simulink model "untitled"  (R2025a)
settings: Solver=VariableStepAuto  StartTime=0.0  StopTime=600  RelTol=1e-3  AbsTol=1e-3  EnableMultiTasking=on
libraries: fl_lib x60, nesl_utility x23, ee_lib x14, slpidlib x4, batteryecm_lib x1, simulink x1
(part 2 of 2)

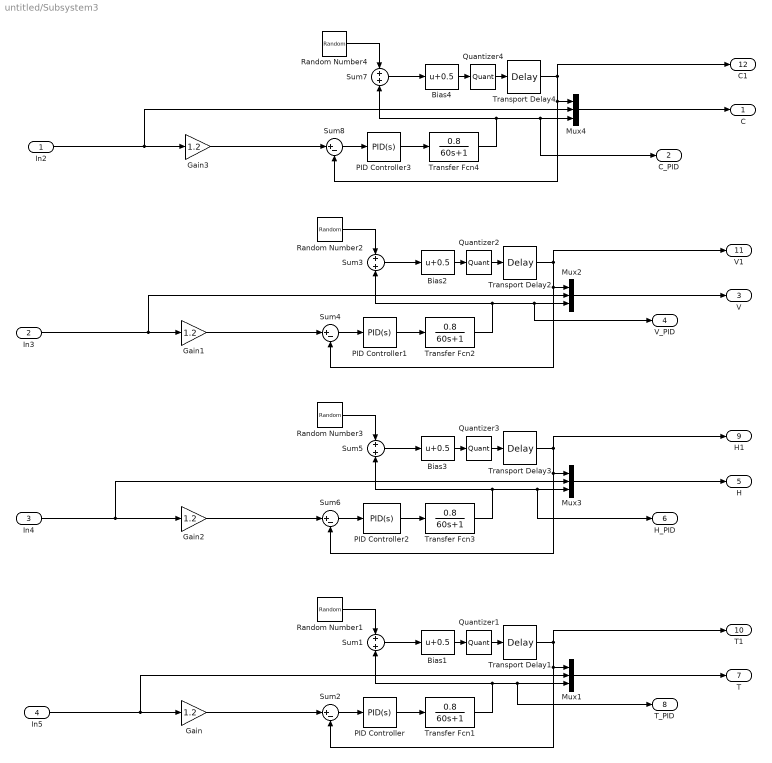
== system untitled/Subsystem3 ==
  In2 : Inport
  In3 : Inport  Port=2
  In4 : Inport  Port=3
  In5 : Inport  Port=4
  Bias{1..4} (4 alike) : Bias  Bias=0.5
  Gain{,1..3} (4 alike) : Gain  Gain=1.2
  Mux{1..4} (4 alike) : Mux  Inputs=3
  PID Controller : slpidlib/PID Controller  Controller=PID  Form=Parallel  TimeDomain=Continuous-time  UseExternalTs=off  SampleTime=-1  IntegratorMethod=Forward Euler  FilterMethod=Forward Euler  ControllerParametersSource=internal  P=2.12001784714755  I=0.0555587280074355  UseKiTs=off  D=0  UseExternalDerivativeSource=off  N=0.0353057614691729  UseFilter=on  TunerSelectOption=Transfer Function Based (PID Tuner App)  InitialConditionSource=internal  InitialConditionForIntegrator=0  InitialConditionForFilter=0  DifferentiatorICPrevScaledInput=0  ExternalReset=none  TrackingMode=off  Kt=1  LimitOutput=off  SatLimitsSource=internal  UpperSaturationLimit=inf  LowerSaturationLimit=-inf  LinearizeAsGain=on  AntiWindupMode=none  Kb=1  LimitIntegrator=off  UpperIntegratorSaturationLimit=inf  LowerIntegratorSaturationLimit=-inf  POutMin=[]  POutMax=[]  IOutMin=[]  IOutMax=[]  DOutMin=[]  DOutMax=[]  NOutMin=[]  NOutMax=[]  SumOutMin=[]  SumOutMax=[]  SaturationOutMin=[]  SaturationOutMax=[]  PParamMin=[]  PParamMax=[]  IParamMin=[]  IParamMax=[]  DParamMin=[]  DParamMax=[]  NParamMin=[]  NParamMax=[]  KbParamMin=[]  KbParamMax=[]  KtParamMin=[]  KtParamMax=[]  KbOutMin=[]  KbOutMax=[]  KtOutMin=[]  KtOutMax=[]  IntegratorOutMin=[]  IntegratorOutMax=[]  FilterOutMin=[]  FilterOutMax=[]  SumI1OutMin=[]  SumI1OutMax=[]  SumI2OutMin=[]  SumI2OutMax=[]  SumI3OutMin=[]  SumI3OutMax=[]  SumI4OutMin=[]  SumI4OutMax=[]  SumDOutMin=[]  SumDOutMax=[]  DifferentiatorOutMin=[]  DifferentiatorOutMax=[]  FilterDiffOutCoefMin=[]  FilterDiffOutCoefMax=[]  ReciprocalOutMin=[]  ReciprocalOutMax=[]  SumDenOutMin=[]  SumDenOutMax=[]  SumNumOutMin=[]  SumNumOutMax=[]  DivideOutMin=[]  DivideOutMax=[]  UdiffTsProdOutMin=[]  UdiffTsProdOutMax=[]  NTsProdOutMin=[]  NTsProdOutMax=[]  UintegralTsProdOutMin=[]  UintegralTsProdOutMax=[]  UngainTsProdOutMin=[]  UngainTsProdOutMax=[]  ClampingZeroOutDataTypeStr=Inherit: Inherit via back propagation  ClampingZeroOutMin=[]  ClampingZeroOutMax=[]  FilterDenConstantOutDataTypeStr=Inherit: Inherit via back propagation  FilterDenConstantOutMin=[]  FilterDenConstantOutMax=[]  PCopyOutDataTypeStr=Inherit: Inherit via back propagation  PCopyOutMin=[]  PCopyOutMax=[]  NCopyOutDataTypeStr=Inherit: Inherit via back propagation  NCopyOutMin=[]  NCopyOutMax=[]  IntegratorContinuousStateAttributes=''  IntegratorStateMustResolveToSignalObject=off  IntegratorRTWStateStorageClass=Auto  FilterContinuousStateAttributes=''  FilterStateMustResolveToSignalObject=off  FilterRTWStateStorageClass=Auto  ParallelPVariant=InternalParameters  IdealPVariant=Disabled  IVariant=InternalParameters  DVariant=InternalParameters  IntegratorVariant=Continuous  SatVariant=Disabled  AWVariant=Passthrough  PCopyVariant=Disabled  TRVariant=Disabled  FdbkBlocksVariant=Forward  IdealPFdbkVariant=Disabled  SatFdbkVariant=Disabled  DerivativeFilterVariant=ContFilter  NVariant=InternalParameters  NCopyVariant=Disabled  FilterICVariant=InternalICsFilter  IntegratorICVariant=InternalICs  ExternalResetVariant=Disabled  TRSumVariant=Passthrough  SumFdbkVariant=Disabled  SumVariant=Sum_PID  TsampFilterVariant=InternalTs  TsampNgainVariant=Passthrough  TsampIntegralVariant=Disabled_SignalSpec  ExternalSaturationOutDataTypeStr=Inherit: Same as second input  DerivativeSourceVariant=ErrorSignal  PreIntVariant=InternalPreInt
  PID Controller1 : slpidlib/PID Controller  Controller=PID  Form=Parallel  TimeDomain=Continuous-time  UseExternalTs=off  SampleTime=-1  IntegratorMethod=Forward Euler  FilterMethod=Forward Euler  ControllerParametersSource=internal  P=2.12001784714755  I=0.0555587280074355  UseKiTs=off  D=0  UseExternalDerivativeSource=off  N=100  UseFilter=on  TunerSelectOption=Transfer Function Based (PID Tuner App)  InitialConditionSource=internal  InitialConditionForIntegrator=0  InitialConditionForFilter=0  DifferentiatorICPrevScaledInput=0  ExternalReset=none  TrackingMode=off  Kt=1  LimitOutput=off  SatLimitsSource=internal  UpperSaturationLimit=inf  LowerSaturationLimit=-inf  LinearizeAsGain=on  AntiWindupMode=none  Kb=1  LimitIntegrator=off  UpperIntegratorSaturationLimit=inf  LowerIntegratorSaturationLimit=-inf  POutMin=[]  POutMax=[]  IOutMin=[]  IOutMax=[]  DOutMin=[]  DOutMax=[]  NOutMin=[]  NOutMax=[]  SumOutMin=[]  SumOutMax=[]  SaturationOutMin=[]  SaturationOutMax=[]  PParamMin=[]  PParamMax=[]  IParamMin=[]  IParamMax=[]  DParamMin=[]  DParamMax=[]  NParamMin=[]  NParamMax=[]  KbParamMin=[]  KbParamMax=[]  KtParamMin=[]  KtParamMax=[]  KbOutMin=[]  KbOutMax=[]  KtOutMin=[]  KtOutMax=[]  IntegratorOutMin=[]  IntegratorOutMax=[]  FilterOutMin=[]  FilterOutMax=[]  SumI1OutMin=[]  SumI1OutMax=[]  SumI2OutMin=[]  SumI2OutMax=[]  SumI3OutMin=[]  SumI3OutMax=[]  SumI4OutMin=[]  SumI4OutMax=[]  SumDOutMin=[]  SumDOutMax=[]  DifferentiatorOutMin=[]  DifferentiatorOutMax=[]  FilterDiffOutCoefMin=[]  FilterDiffOutCoefMax=[]  ReciprocalOutMin=[]  ReciprocalOutMax=[]  SumDenOutMin=[]  SumDenOutMax=[]  SumNumOutMin=[]  SumNumOutMax=[]  DivideOutMin=[]  DivideOutMax=[]  UdiffTsProdOutMin=[]  UdiffTsProdOutMax=[]  NTsProdOutMin=[]  NTsProdOutMax=[]  UintegralTsProdOutMin=[]  UintegralTsProdOutMax=[]  UngainTsProdOutMin=[]  UngainTsProdOutMax=[]  ClampingZeroOutDataTypeStr=Inherit: Inherit via back propagation  ClampingZeroOutMin=[]  ClampingZeroOutMax=[]  FilterDenConstantOutDataTypeStr=Inherit: Inherit via back propagation  FilterDenConstantOutMin=[]  FilterDenConstantOutMax=[]  PCopyOutDataTypeStr=Inherit: Inherit via back propagation  PCopyOutMin=[]  PCopyOutMax=[]  NCopyOutDataTypeStr=Inherit: Inherit via back propagation  NCopyOutMin=[]  NCopyOutMax=[]  IntegratorContinuousStateAttributes=''  IntegratorStateMustResolveToSignalObject=off  IntegratorRTWStateStorageClass=Auto  FilterContinuousStateAttributes=''  FilterStateMustResolveToSignalObject=off  FilterRTWStateStorageClass=Auto  ParallelPVariant=InternalParameters  IdealPVariant=Disabled  IVariant=InternalParameters  DVariant=InternalParameters  IntegratorVariant=Continuous  SatVariant=Disabled  AWVariant=Passthrough  PCopyVariant=Disabled  TRVariant=Disabled  FdbkBlocksVariant=Forward  IdealPFdbkVariant=Disabled  SatFdbkVariant=Disabled  DerivativeFilterVariant=ContFilter  NVariant=InternalParameters  NCopyVariant=Disabled  FilterICVariant=InternalICsFilter  IntegratorICVariant=InternalICs  ExternalResetVariant=Disabled  TRSumVariant=Passthrough  SumFdbkVariant=Disabled  SumVariant=Sum_PID  TsampFilterVariant=InternalTs  TsampNgainVariant=Passthrough  TsampIntegralVariant=Disabled_SignalSpec  ExternalSaturationOutDataTypeStr=Inherit: Same as second input  DerivativeSourceVariant=ErrorSignal  PreIntVariant=InternalPreInt
  PID Controller2 : slpidlib/PID Controller  Controller=PID  Form=Parallel  TimeDomain=Continuous-time  UseExternalTs=off  SampleTime=-1  IntegratorMethod=Forward Euler  FilterMethod=Forward Euler  ControllerParametersSource=internal  P=2.12001784714755  I=0.0555587280074355  UseKiTs=off  D=0  UseExternalDerivativeSource=off  N=100  UseFilter=on  TunerSelectOption=Transfer Function Based (PID Tuner App)  InitialConditionSource=internal  InitialConditionForIntegrator=0  InitialConditionForFilter=0  DifferentiatorICPrevScaledInput=0  ExternalReset=none  TrackingMode=off  Kt=1  LimitOutput=off  SatLimitsSource=internal  UpperSaturationLimit=inf  LowerSaturationLimit=-inf  LinearizeAsGain=on  AntiWindupMode=none  Kb=1  LimitIntegrator=off  UpperIntegratorSaturationLimit=inf  LowerIntegratorSaturationLimit=-inf  POutMin=[]  POutMax=[]  IOutMin=[]  IOutMax=[]  DOutMin=[]  DOutMax=[]  NOutMin=[]  NOutMax=[]  SumOutMin=[]  SumOutMax=[]  SaturationOutMin=[]  SaturationOutMax=[]  PParamMin=[]  PParamMax=[]  IParamMin=[]  IParamMax=[]  DParamMin=[]  DParamMax=[]  NParamMin=[]  NParamMax=[]  KbParamMin=[]  KbParamMax=[]  KtParamMin=[]  KtParamMax=[]  KbOutMin=[]  KbOutMax=[]  KtOutMin=[]  KtOutMax=[]  IntegratorOutMin=[]  IntegratorOutMax=[]  FilterOutMin=[]  FilterOutMax=[]  SumI1OutMin=[]  SumI1OutMax=[]  SumI2OutMin=[]  SumI2OutMax=[]  SumI3OutMin=[]  SumI3OutMax=[]  SumI4OutMin=[]  SumI4OutMax=[]  SumDOutMin=[]  SumDOutMax=[]  DifferentiatorOutMin=[]  DifferentiatorOutMax=[]  FilterDiffOutCoefMin=[]  FilterDiffOutCoefMax=[]  ReciprocalOutMin=[]  ReciprocalOutMax=[]  SumDenOutMin=[]  SumDenOutMax=[]  SumNumOutMin=[]  SumNumOutMax=[]  DivideOutMin=[]  DivideOutMax=[]  UdiffTsProdOutMin=[]  UdiffTsProdOutMax=[]  NTsProdOutMin=[]  NTsProdOutMax=[]  UintegralTsProdOutMin=[]  UintegralTsProdOutMax=[]  UngainTsProdOutMin=[]  UngainTsProdOutMax=[]  ClampingZeroOutDataTypeStr=Inherit: Inherit via back propagation  ClampingZeroOutMin=[]  ClampingZeroOutMax=[]  FilterDenConstantOutDataTypeStr=Inherit: Inherit via back propagation  FilterDenConstantOutMin=[]  FilterDenConstantOutMax=[]  PCopyOutDataTypeStr=Inherit: Inherit via back propagation  PCopyOutMin=[]  PCopyOutMax=[]  NCopyOutDataTypeStr=Inherit: Inherit via back propagation  NCopyOutMin=[]  NCopyOutMax=[]  IntegratorContinuousStateAttributes=''  IntegratorStateMustResolveToSignalObject=off  IntegratorRTWStateStorageClass=Auto  FilterContinuousStateAttributes=''  FilterStateMustResolveToSignalObject=off  FilterRTWStateStorageClass=Auto  ParallelPVariant=InternalParameters  IdealPVariant=Disabled  IVariant=InternalParameters  DVariant=InternalParameters  IntegratorVariant=Continuous  SatVariant=Disabled  AWVariant=Passthrough  PCopyVariant=Disabled  TRVariant=Disabled  FdbkBlocksVariant=Forward  IdealPFdbkVariant=Disabled  SatFdbkVariant=Disabled  DerivativeFilterVariant=ContFilter  NVariant=InternalParameters  NCopyVariant=Disabled  FilterICVariant=InternalICsFilter  IntegratorICVariant=InternalICs  ExternalResetVariant=Disabled  TRSumVariant=Passthrough  SumFdbkVariant=Disabled  SumVariant=Sum_PID  TsampFilterVariant=InternalTs  TsampNgainVariant=Passthrough  TsampIntegralVariant=Disabled_SignalSpec  ExternalSaturationOutDataTypeStr=Inherit: Same as second input  DerivativeSourceVariant=ErrorSignal  PreIntVariant=InternalPreInt
  PID Controller3 : slpidlib/PID Controller  Controller=PID  Form=Parallel  TimeDomain=Continuous-time  UseExternalTs=off  SampleTime=-1  IntegratorMethod=Forward Euler  FilterMethod=Forward Euler  ControllerParametersSource=internal  P=2.12001784714755  I=0.0425233068957785  UseKiTs=off  D=8.52577757434395  UseExternalDerivativeSource=off  N=0.0510689208285348  UseFilter=on  TunerSelectOption=Transfer Function Based (PID Tuner App)  InitialConditionSource=internal  InitialConditionForIntegrator=0  InitialConditionForFilter=0  DifferentiatorICPrevScaledInput=0  ExternalReset=none  TrackingMode=off  Kt=1  LimitOutput=off  SatLimitsSource=internal  UpperSaturationLimit=inf  LowerSaturationLimit=-inf  LinearizeAsGain=on  AntiWindupMode=none  Kb=1  LimitIntegrator=off  UpperIntegratorSaturationLimit=inf  LowerIntegratorSaturationLimit=-inf  POutMin=[]  POutMax=[]  IOutMin=[]  IOutMax=[]  DOutMin=[]  DOutMax=[]  NOutMin=[]  NOutMax=[]  SumOutMin=[]  SumOutMax=[]  SaturationOutMin=[]  SaturationOutMax=[]  PParamMin=[]  PParamMax=[]  IParamMin=[]  IParamMax=[]  DParamMin=[]  DParamMax=[]  NParamMin=[]  NParamMax=[]  KbParamMin=[]  KbParamMax=[]  KtParamMin=[]  KtParamMax=[]  KbOutMin=[]  KbOutMax=[]  KtOutMin=[]  KtOutMax=[]  IntegratorOutMin=[]  IntegratorOutMax=[]  FilterOutMin=[]  FilterOutMax=[]  SumI1OutMin=[]  SumI1OutMax=[]  SumI2OutMin=[]  SumI2OutMax=[]  SumI3OutMin=[]  SumI3OutMax=[]  SumI4OutMin=[]  SumI4OutMax=[]  SumDOutMin=[]  SumDOutMax=[]  DifferentiatorOutMin=[]  DifferentiatorOutMax=[]  FilterDiffOutCoefMin=[]  FilterDiffOutCoefMax=[]  ReciprocalOutMin=[]  ReciprocalOutMax=[]  SumDenOutMin=[]  SumDenOutMax=[]  SumNumOutMin=[]  SumNumOutMax=[]  DivideOutMin=[]  DivideOutMax=[]  UdiffTsProdOutMin=[]  UdiffTsProdOutMax=[]  NTsProdOutMin=[]  NTsProdOutMax=[]  UintegralTsProdOutMin=[]  UintegralTsProdOutMax=[]  UngainTsProdOutMin=[]  UngainTsProdOutMax=[]  ClampingZeroOutDataTypeStr=Inherit: Inherit via back propagation  ClampingZeroOutMin=[]  ClampingZeroOutMax=[]  FilterDenConstantOutDataTypeStr=Inherit: Inherit via back propagation  FilterDenConstantOutMin=[]  FilterDenConstantOutMax=[]  PCopyOutDataTypeStr=Inherit: Inherit via back propagation  PCopyOutMin=[]  PCopyOutMax=[]  NCopyOutDataTypeStr=Inherit: Inherit via back propagation  NCopyOutMin=[]  NCopyOutMax=[]  IntegratorContinuousStateAttributes=''  IntegratorStateMustResolveToSignalObject=off  IntegratorRTWStateStorageClass=Auto  FilterContinuousStateAttributes=''  FilterStateMustResolveToSignalObject=off  FilterRTWStateStorageClass=Auto  ParallelPVariant=InternalParameters  IdealPVariant=Disabled  IVariant=InternalParameters  DVariant=InternalParameters  IntegratorVariant=Continuous  SatVariant=Disabled  AWVariant=Passthrough  PCopyVariant=Disabled  TRVariant=Disabled  FdbkBlocksVariant=Forward  IdealPFdbkVariant=Disabled  SatFdbkVariant=Disabled  DerivativeFilterVariant=ContFilter  NVariant=InternalParameters  NCopyVariant=Disabled  FilterICVariant=InternalICsFilter  IntegratorICVariant=InternalICs  ExternalResetVariant=Disabled  TRSumVariant=Passthrough  SumFdbkVariant=Disabled  SumVariant=Sum_PID  TsampFilterVariant=InternalTs  TsampNgainVariant=Passthrough  TsampIntegralVariant=Disabled_SignalSpec  ExternalSaturationOutDataTypeStr=Inherit: Same as second input  DerivativeSourceVariant=ErrorSignal  PreIntVariant=InternalPreInt
  Quantizer{1..4} (4 alike) : Quantizer  QuantizationInterval=0.390625
  Random Number{1..4} (4 alike) : RandomNumber  Variance=0.1*0.1  SampleTime=1
  Sum{1,3,5,7} (4 alike) : Sum
  Sum{2,4,6,8} (4 alike) : Sum  Inputs=|+-
  Transfer Fcn{1..4} (4 alike) : TransferFcn  Numerator=[0.8]  Denominator=[60 1]
  Transport Delay1 : TransportDelay  DelayTime=0.1
  Transport Delay2 : TransportDelay  DelayTime=0.1
  Transport Delay3 : TransportDelay  DelayTime=0.1
  Transport Delay4 : TransportDelay  DelayTime=0.1  BufferSize=512
  C : Outport
  C_PID : Outport  Port=2
  V : Outport  Port=3
  V_PID : Outport  Port=4
  H : Outport  Port=5
  H_PID : Outport  Port=6
  T : Outport  Port=7
  T_PID : Outport  Port=8
  H1 : Outport  Port=9
  T1 : Outport  Port=10
  V1 : Outport  Port=11
  C1 : Outport  Port=12
  wires:
  Transfer Fcn1/1 -> T_PID/1, Mux1/3, Sum1/2
  In5/1 -> Gain/1, Mux1/2
  Sum2/1 -> PID Controller/1
  PID Controller/1 -> Transfer Fcn1/1
  Sum1/1 -> Bias1/1
  Transport Delay1/1 -> T1/1, Sum2/2, Mux1/1
  Bias1/1 -> Quantizer1/1
  Quantizer1/1 -> Transport Delay1/1
  Mux1/1 -> T/1
  Random Number1/1 -> Sum1/1
  Quantizer2/1 -> Transport Delay2/1
  Bias2/1 -> Quantizer2/1
  Mux2/1 -> V/1
  Sum3/1 -> Bias2/1
  PID Controller1/1 -> Transfer Fcn2/1
  Random Number2/1 -> Sum3/1
  Sum4/1 -> PID Controller1/1
  Transfer Fcn2/1 -> V_PID/1, Mux2/3, Sum3/2
  Transport Delay2/1 -> V1/1, Sum4/2, Mux2/1
  Quantizer3/1 -> Transport Delay3/1
  Bias3/1 -> Quantizer3/1
  Mux3/1 -> H/1
  Sum5/1 -> Bias3/1
  PID Controller2/1 -> Transfer Fcn3/1
  Random Number3/1 -> Sum5/1
  Sum6/1 -> PID Controller2/1
  Transfer Fcn3/1 -> H_PID/1, Mux3/3, Sum5/2
  Transport Delay3/1 -> H1/1, Sum6/2, Mux3/1
  In2/1 -> Mux4/2, Gain3/1
  Quantizer4/1 -> Transport Delay4/1
  Bias4/1 -> Quantizer4/1
  Mux4/1 -> C/1
  Sum7/1 -> Bias4/1
  PID Controller3/1 -> Transfer Fcn4/1
  Random Number4/1 -> Sum7/1
  Sum8/1 -> PID Controller3/1
  Transfer Fcn4/1 -> C_PID/1, Mux4/3, Sum7/2
  Transport Delay4/1 -> C1/1, Sum8/2, Mux4/1
  Gain3/1 -> Sum8/1
  Gain2/1 -> Sum6/1
  Gain1/1 -> Sum4/1
  Gain/1 -> Sum2/1
  In4/1 -> Mux3/2, Gain2/1
  In3/1 -> Mux2/2, Gain1/1

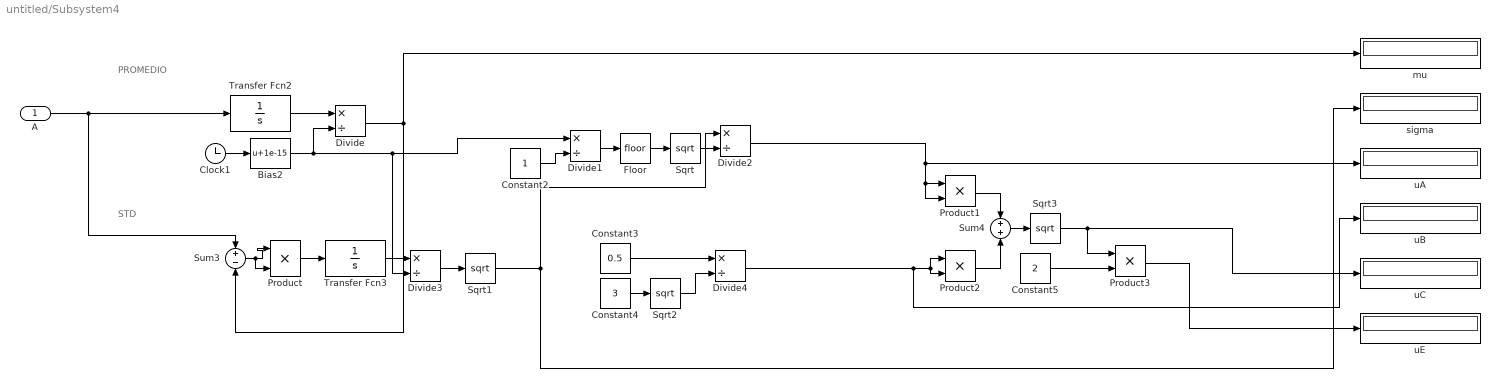
== system untitled/Subsystem4 ==
  note: PROMEDIO
  note: STD
  A : Inport
  Bias2 : Bias  Bias=1e-15  SaturateOnIntegerOverflow=off
  Clock1 : Clock
  Constant2 : Constant
  Constant3 : Constant  Value=0.5
  Constant4 : Constant  Value=3
  Constant5 : Constant  Value=2
  Divide{,1..4} (5 alike) : Product  Inputs=*/
  Floor : Rounding
  Product{,1..3} (4 alike) : Product
  Sqrt{,1..3} (4 alike) : Sqrt
  Sum3 : Sum  Inputs=+-
  Sum4 : Sum
  Transfer Fcn2 : TransferFcn  Denominator=[1 0]
  Transfer Fcn3 : TransferFcn  Denominator=[1 0]
  mu : Display
  sigma : Display
  uA : Display
  uB : Display
  uC : Display
  uE : Display
  wires:
  Divide4/1 -> uB/1, Product2/1, Product2/2
  Sqrt/1 -> Divide2/2
  Divide2/1 -> Product1/2, Product1/1, uA/1
  Transfer Fcn3/1 -> Divide3/1
  A/1 -> Sum3/1, Transfer Fcn2/1
  Sqrt2/1 -> Divide4/2
  Bias2/1 -> Divide3/2, Divide1/1, Divide/2
  Divide1/1 -> Floor/1
  Divide/1 -> Sum3/2, mu/1
  Constant5/1 -> Product3/2
  Sqrt3/1 -> uC/1, Product3/1
  Sqrt1/1 -> sigma/1, Divide2/1
  Floor/1 -> Sqrt/1
  Divide3/1 -> Sqrt1/1
  Product1/1 -> Sum4/1
  Constant3/1 -> Divide4/1
  Product/1 -> Transfer Fcn3/1
  Product2/1 -> Sum4/2
  Constant2/1 -> Divide1/2
  Clock1/1 -> Bias2/1
  Product3/1 -> uE/1
  Transfer Fcn2/1 -> Divide/1
  Sum3/1 -> Product/1, Product/2
  Constant4/1 -> Sqrt2/1
  Sum4/1 -> Sqrt3/1

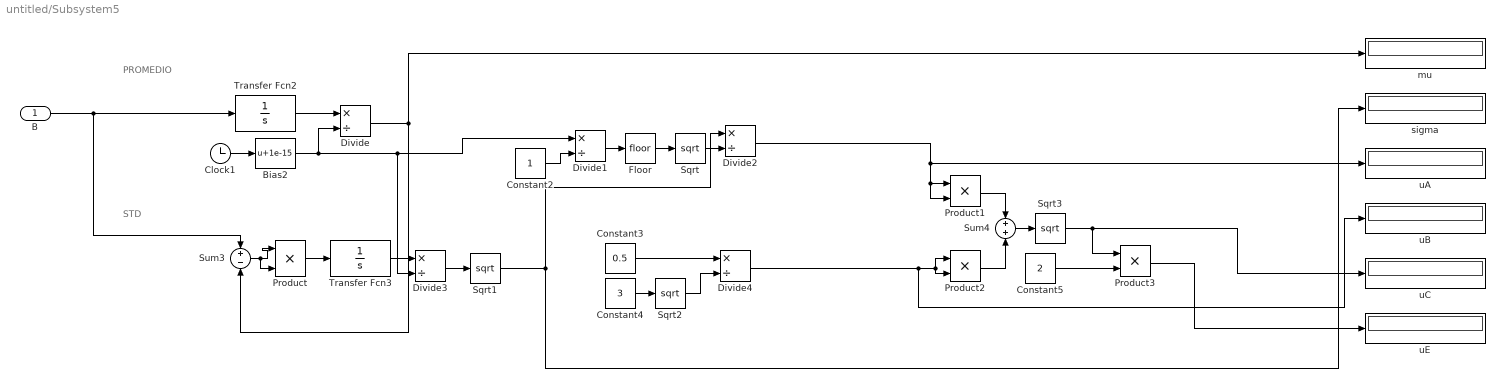
== system untitled/Subsystem5 ==
  note: STD
  note: PROMEDIO
  B : Inport
  Bias2 : Bias  Bias=1e-15  SaturateOnIntegerOverflow=off
  Clock1 : Clock
  Constant2 : Constant
  Constant3 : Constant  Value=0.5
  Constant4 : Constant  Value=3
  Constant5 : Constant  Value=2
  Divide{,1..4} (5 alike) : Product  Inputs=*/
  Floor : Rounding
  Product{,1..3} (4 alike) : Product
  Sqrt{,1..3} (4 alike) : Sqrt
  Sum3 : Sum  Inputs=+-
  Sum4 : Sum
  Transfer Fcn2 : TransferFcn  Denominator=[1 0]
  Transfer Fcn3 : TransferFcn  Denominator=[1 0]
  mu : Display
  sigma : Display
  uA : Display
  uB : Display
  uC : Display
  uE : Display
  wires:
  B/1 -> Sum3/1, Transfer Fcn2/1
  Sum3/1 -> Product/1, Product/2
  Divide4/1 -> uB/1, Product2/1, Product2/2
  Sum4/1 -> Sqrt3/1
  Sqrt1/1 -> sigma/1, Divide2/1
  Constant4/1 -> Sqrt2/1
  Clock1/1 -> Bias2/1
  Transfer Fcn2/1 -> Divide/1
  Divide3/1 -> Sqrt1/1
  Floor/1 -> Sqrt/1
  Product1/1 -> Sum4/1
  Constant5/1 -> Product3/2
  Constant3/1 -> Divide4/1
  Constant2/1 -> Divide1/2
  Product2/1 -> Sum4/2
  Transfer Fcn3/1 -> Divide3/1
  Sqrt3/1 -> uC/1, Product3/1
  Product3/1 -> uE/1
  Bias2/1 -> Divide3/2, Divide1/1, Divide/2
  Divide1/1 -> Floor/1
  Sqrt2/1 -> Divide4/2
  Divide/1 -> Sum3/2, mu/1
  Divide2/1 -> Product1/2, Product1/1, uA/1
  Sqrt/1 -> Divide2/2
  Product/1 -> Transfer Fcn3/1

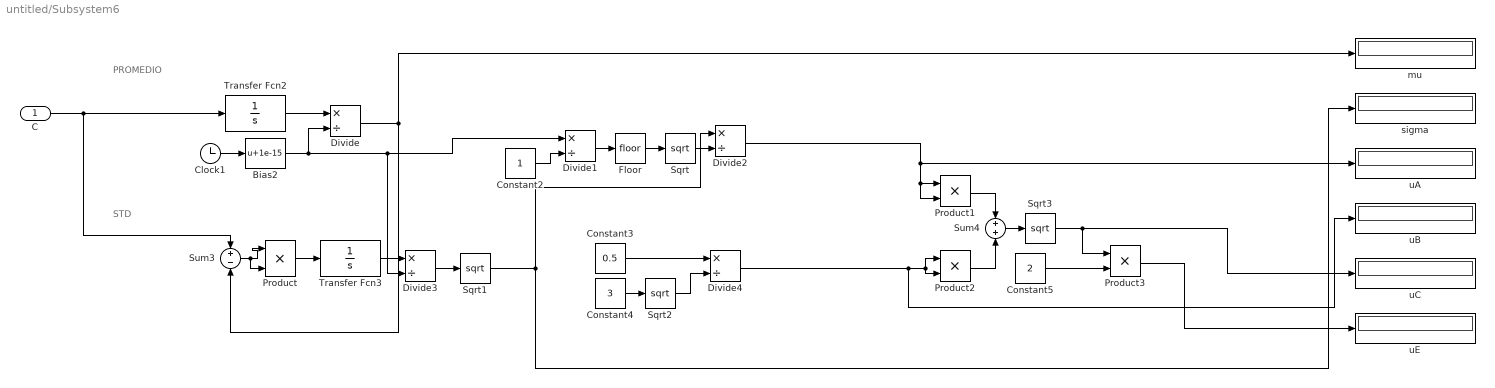
== system untitled/Subsystem6 ==
  note: STD
  note: PROMEDIO
  C : Inport
  Bias2 : Bias  Bias=1e-15  SaturateOnIntegerOverflow=off
  Clock1 : Clock
  Constant2 : Constant
  Constant3 : Constant  Value=0.5
  Constant4 : Constant  Value=3
  Constant5 : Constant  Value=2
  Divide{,1..4} (5 alike) : Product  Inputs=*/
  Floor : Rounding
  Product{,1..3} (4 alike) : Product
  Sqrt{,1..3} (4 alike) : Sqrt
  Sum3 : Sum  Inputs=+-
  Sum4 : Sum
  Transfer Fcn2 : TransferFcn  Denominator=[1 0]
  Transfer Fcn3 : TransferFcn  Denominator=[1 0]
  mu : Display
  sigma : Display
  uA : Display
  uB : Display
  uC : Display
  uE : Display
  wires:
  C/1 -> Sum3/1, Transfer Fcn2/1
  Sum3/1 -> Product/1, Product/2
  Divide4/1 -> uB/1, Product2/1, Product2/2
  Sum4/1 -> Sqrt3/1
  Sqrt1/1 -> sigma/1, Divide2/1
  Constant4/1 -> Sqrt2/1
  Clock1/1 -> Bias2/1
  Transfer Fcn2/1 -> Divide/1
  Divide3/1 -> Sqrt1/1
  Floor/1 -> Sqrt/1
  Product1/1 -> Sum4/1
  Constant5/1 -> Product3/2
  Constant3/1 -> Divide4/1
  Constant2/1 -> Divide1/2
  Product2/1 -> Sum4/2
  Transfer Fcn3/1 -> Divide3/1
  Sqrt3/1 -> uC/1, Product3/1
  Product3/1 -> uE/1
  Bias2/1 -> Divide3/2, Divide1/1, Divide/2
  Divide1/1 -> Floor/1
  Sqrt2/1 -> Divide4/2
  Divide/1 -> Sum3/2, mu/1
  Divide2/1 -> Product1/2, Product1/1, uA/1
  Sqrt/1 -> Divide2/2
  Product/1 -> Transfer Fcn3/1

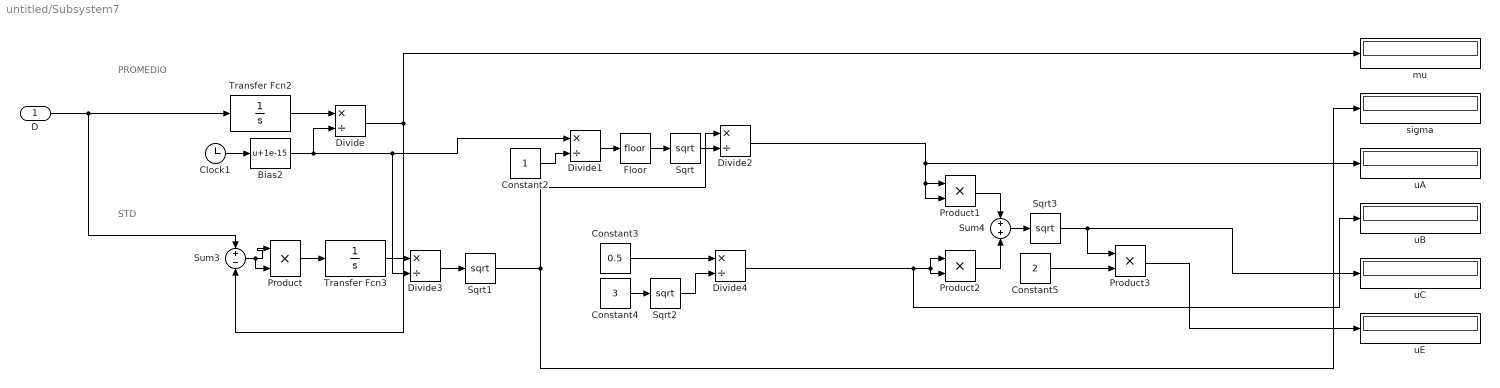
== system untitled/Subsystem7 ==
  note: STD
  note: PROMEDIO
  D : Inport
  Bias2 : Bias  Bias=1e-15  SaturateOnIntegerOverflow=off
  Clock1 : Clock
  Constant2 : Constant
  Constant3 : Constant  Value=0.5
  Constant4 : Constant  Value=3
  Constant5 : Constant  Value=2
  Divide{,1..4} (5 alike) : Product  Inputs=*/
  Floor : Rounding
  Product{,1..3} (4 alike) : Product
  Sqrt{,1..3} (4 alike) : Sqrt
  Sum3 : Sum  Inputs=+-
  Sum4 : Sum
  Transfer Fcn2 : TransferFcn  Denominator=[1 0]
  Transfer Fcn3 : TransferFcn  Denominator=[1 0]
  mu : Display
  sigma : Display
  uA : Display
  uB : Display
  uC : Display
  uE : Display
  wires:
  D/1 -> Sum3/1, Transfer Fcn2/1
  Sum3/1 -> Product/1, Product/2
  Divide4/1 -> uB/1, Product2/1, Product2/2
  Sum4/1 -> Sqrt3/1
  Sqrt1/1 -> sigma/1, Divide2/1
  Constant4/1 -> Sqrt2/1
  Clock1/1 -> Bias2/1
  Transfer Fcn2/1 -> Divide/1
  Divide3/1 -> Sqrt1/1
  Floor/1 -> Sqrt/1
  Product1/1 -> Sum4/1
  Constant5/1 -> Product3/2
  Constant3/1 -> Divide4/1
  Constant2/1 -> Divide1/2
  Product2/1 -> Sum4/2
  Transfer Fcn3/1 -> Divide3/1
  Sqrt3/1 -> uC/1, Product3/1
  Product3/1 -> uE/1
  Bias2/1 -> Divide3/2, Divide1/1, Divide/2
  Divide1/1 -> Floor/1
  Sqrt2/1 -> Divide4/2
  Divide/1 -> Sum3/2, mu/1
  Divide2/1 -> Product1/2, Product1/1, uA/1
  Sqrt/1 -> Divide2/2
  Product/1 -> Transfer Fcn3/1

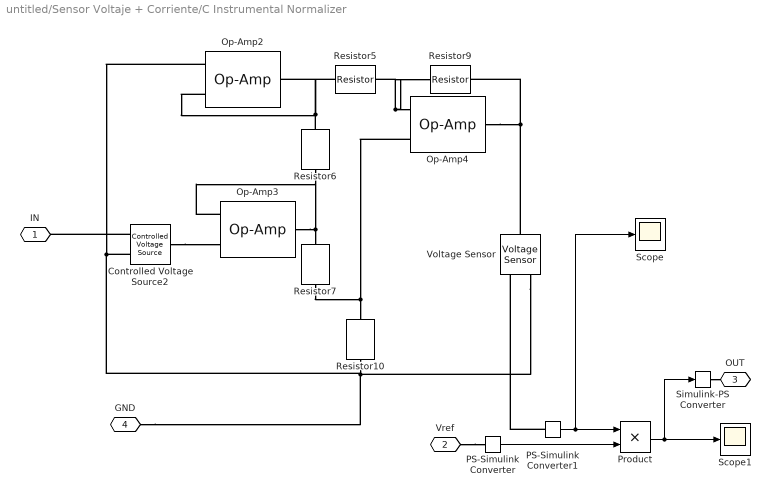
== system untitled/Sensor Voltaje + Corriente/C Instrumental Normalizer ==
  Controlled Voltage Source2 : fl_lib/Electrical/Electrical Sources/Controlled Voltage Source
  Op-Amp2 : fl_lib/Electrical/Electrical Elements/Op-Amp  outI_specify=off  outI_priority=None  outI=0 A  outI_nominal_specify=on  outI_nominal_value=1  outI_nominal_unit=A
  Op-Amp3 : fl_lib/Electrical/Electrical Elements/Op-Amp  outI_specify=off  outI_priority=None  outI=0 A  outI_nominal_specify=on  outI_nominal_value=1  outI_nominal_unit=A
  Op-Amp4 : fl_lib/Electrical/Electrical Elements/Op-Amp  outI_specify=off  outI_priority=None  outI=0 A  outI_nominal_specify=on  outI_nominal_value=1  outI_nominal_unit=A
  PS-Simulink Converter : nesl_utility/PS-Simulink Converter  PhysicalDomain=network_engine_domain  SubClassName=ps_output  LeftPortType=input  RightPortType=output  PseudoPeriodic=off  Frequencies=[]  VectorFormat=inherit  Unit=inherit  AffineConversion=off
  PS-Simulink Converter1 : nesl_utility/PS-Simulink Converter  PhysicalDomain=network_engine_domain  SubClassName=ps_output  LeftPortType=input  RightPortType=output  PseudoPeriodic=off  Frequencies=[]  VectorFormat=inherit  Unit=inherit  AffineConversion=off
  Product : Product
  Resistor10 : fl_lib/Electrical/Electrical Elements/Resistor  R=660 Ohm  i_specify=off  i_priority=None  i=0 A  i_nominal_specify=off  i_nominal_value=1  i_nominal_unit=A  v_specify=off  v_priority=None  v=0 V  v_nominal_specify=off  v_nominal_value=1  v_nominal_unit=V
  Resistor5 : fl_lib/Electrical/Electrical Elements/Resistor  R=66 kOhm  i_specify=off  i_priority=None  i=0 A  i_nominal_specify=off  i_nominal_value=1  i_nominal_unit=A  v_specify=off  v_priority=None  v=0 V  v_nominal_specify=off  v_nominal_value=1  v_nominal_unit=V
  Resistor6 : fl_lib/Electrical/Electrical Elements/Resistor  R=33 kOhm  i_specify=off  i_priority=None  i=0 A  i_nominal_specify=off  i_nominal_value=1  i_nominal_unit=A  v_specify=off  v_priority=None  v=0 V  v_nominal_specify=off  v_nominal_value=1  v_nominal_unit=V
  Resistor7 : fl_lib/Electrical/Electrical Elements/Resistor  R=66 kOhm  i_specify=off  i_priority=None  i=0 A  i_nominal_specify=off  i_nominal_value=1  i_nominal_unit=A  v_specify=off  v_priority=None  v=0 V  v_nominal_specify=off  v_nominal_value=1  v_nominal_unit=V
  Resistor9 : fl_lib/Electrical/Electrical Elements/Resistor  R=660 Ohm  i_specify=off  i_priority=None  i=0 A  i_nominal_specify=off  i_nominal_value=1  i_nominal_unit=A  v_specify=off  v_priority=None  v=0 V  v_nominal_specify=off  v_nominal_value=1  v_nominal_unit=V
  Scope : Scope
      settings: ActiveDisplayYMinimum=-0.23873506450497317  ActiveDisplayYMaximum=3.7811184866173342
  Scope1 : Scope
      settings: ActiveDisplayYMinimum=-0.23201568063528288  ActiveDisplayYMaximum=5.0745797296535642
  Simulink-PS Converter : nesl_utility/Simulink-PS Converter  PhysicalDomain=network_engine_domain  SubClassName=ps_input  LeftPortType=input  RightPortType=output  PseudoPeriodic=off  Frequencies=[]  NoiseDistribution=none  NoiseParameters=[]  Unit=1  AffineConversion=off  FilteringAndDerivatives=provide  SimscapeFilterOrder=1  InputFilterTimeConstant=0.001  UdotUserProvided=0
  Voltage Sensor : fl_lib/Electrical/Electrical Sensors/Voltage Sensor
  IN : PMIOPort  Side=Left
  Vref : PMIOPort  Port=2  Side=Left
  OUT : PMIOPort  Port=3  Side=Left
  GND : PMIOPort  Port=4  Side=Right
  wires:
  PS-Simulink Converter/1 -> Product/2
  PS-Simulink Converter1/1 -> Scope/1, Product/1
  Product/1 -> Simulink-PS Converter/1, Scope1/1
  connections:
  Op-Amp4/LConn1 -- Resistor10/LConn1 -- Resistor7/RConn1
  Controlled Voltage Source2/LConn1 -- Op-Amp3/LConn1
  Resistor10/RConn1 -- GND/RConn1 -- Op-Amp2/LConn1 -- Controlled Voltage Source2/RConn2 -- Voltage Sensor/RConn2
  Op-Amp4/LConn2 -- Resistor9/LConn1 -- Resistor5/LConn1
  Op-Amp4/RConn1 -- Resistor9/RConn1 -- Voltage Sensor/LConn1
  Op-Amp2/LConn2 -- Resistor6/LConn1 -- Resistor5/RConn1 -- Op-Amp2/RConn1
  Op-Amp3/RConn1 -- Resistor7/LConn1 -- Op-Amp3/LConn2 -- Resistor6/RConn1
  Controlled Voltage Source2/RConn1 -- IN/RConn1
  Vref/RConn1 -- PS-Simulink Converter/LConn1
  PS-Simulink Converter1/LConn1 -- Voltage Sensor/RConn1
  Simulink-PS Converter/RConn1 -- OUT/RConn1

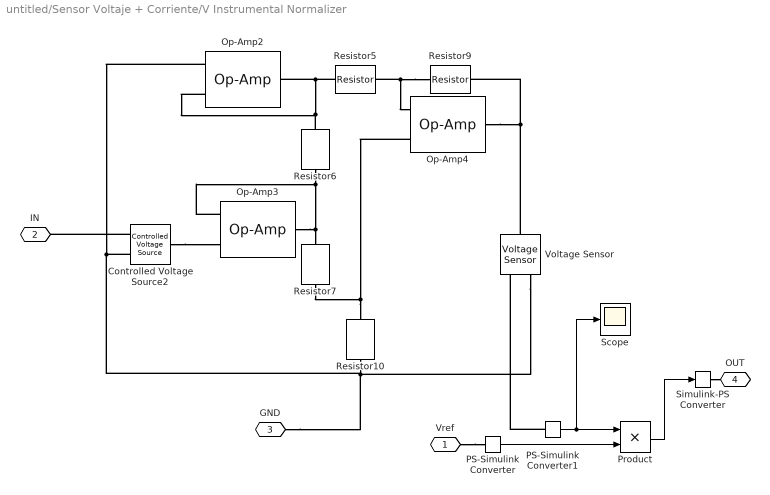
== system untitled/Sensor Voltaje + Corriente/V Instrumental Normalizer ==
  Controlled Voltage Source2 : fl_lib/Electrical/Electrical Sources/Controlled Voltage Source
  Op-Amp2 : fl_lib/Electrical/Electrical Elements/Op-Amp  outI_specify=off  outI_priority=None  outI=0 A  outI_nominal_specify=on  outI_nominal_value=1  outI_nominal_unit=A
  Op-Amp3 : fl_lib/Electrical/Electrical Elements/Op-Amp  outI_specify=off  outI_priority=None  outI=0 A  outI_nominal_specify=on  outI_nominal_value=1  outI_nominal_unit=A
  Op-Amp4 : fl_lib/Electrical/Electrical Elements/Op-Amp  outI_specify=off  outI_priority=None  outI=0 A  outI_nominal_specify=on  outI_nominal_value=1  outI_nominal_unit=A
  PS-Simulink Converter : nesl_utility/PS-Simulink Converter  PhysicalDomain=network_engine_domain  SubClassName=ps_output  LeftPortType=input  RightPortType=output  PseudoPeriodic=off  Frequencies=[]  VectorFormat=inherit  Unit=inherit  AffineConversion=off
  PS-Simulink Converter1 : nesl_utility/PS-Simulink Converter  PhysicalDomain=network_engine_domain  SubClassName=ps_output  LeftPortType=input  RightPortType=output  PseudoPeriodic=off  Frequencies=[]  VectorFormat=inherit  Unit=inherit  AffineConversion=off
  Product : Product
  Resistor10 : fl_lib/Electrical/Electrical Elements/Resistor  R=6.6 Ohm  i_specify=off  i_priority=None  i=0 A  i_nominal_specify=off  i_nominal_value=1  i_nominal_unit=A  v_specify=off  v_priority=None  v=0 V  v_nominal_specify=off  v_nominal_value=1  v_nominal_unit=V
  Resistor5 : fl_lib/Electrical/Electrical Elements/Resistor  R=6.6 kOhm  i_specify=off  i_priority=None  i=0 A  i_nominal_specify=off  i_nominal_value=1  i_nominal_unit=A  v_specify=off  v_priority=None  v=0 V  v_nominal_specify=off  v_nominal_value=1  v_nominal_unit=V
  Resistor6 : fl_lib/Electrical/Electrical Elements/Resistor  R=3.3 kOhm  i_specify=off  i_priority=None  i=0 A  i_nominal_specify=off  i_nominal_value=1  i_nominal_unit=A  v_specify=off  v_priority=None  v=0 V  v_nominal_specify=off  v_nominal_value=1  v_nominal_unit=V
  Resistor7 : fl_lib/Electrical/Electrical Elements/Resistor  R=6.6 kOhm  i_specify=off  i_priority=None  i=0 A  i_nominal_specify=off  i_nominal_value=1  i_nominal_unit=A  v_specify=off  v_priority=None  v=0 V  v_nominal_specify=off  v_nominal_value=1  v_nominal_unit=V
  Resistor9 : fl_lib/Electrical/Electrical Elements/Resistor  R=6.6 Ohm  i_specify=off  i_priority=None  i=0 A  i_nominal_specify=off  i_nominal_value=1  i_nominal_unit=A  v_specify=off  v_priority=None  v=0 V  v_nominal_specify=off  v_nominal_value=1  v_nominal_unit=V
  Scope : Scope
      settings: ActiveDisplayYMinimum=-1  ActiveDisplayYMaximum=1
  Simulink-PS Converter : nesl_utility/Simulink-PS Converter  PhysicalDomain=network_engine_domain  SubClassName=ps_input  LeftPortType=input  RightPortType=output  PseudoPeriodic=off  Frequencies=[]  NoiseDistribution=none  NoiseParameters=[]  Unit=1  AffineConversion=off  FilteringAndDerivatives=provide  SimscapeFilterOrder=1  InputFilterTimeConstant=0.001  UdotUserProvided=0
  Voltage Sensor : fl_lib/Electrical/Electrical Sensors/Voltage Sensor
  Vref : PMIOPort  Side=Left
  IN : PMIOPort  Port=2  Side=Left
  GND : PMIOPort  Port=3  Side=Left
  OUT : PMIOPort  Port=4  Side=Right
  wires:
  PS-Simulink Converter/1 -> Product/2
  PS-Simulink Converter1/1 -> Scope/1, Product/1
  Product/1 -> Simulink-PS Converter/1
  connections:
  Resistor10/LConn1 -- Op-Amp4/LConn1 -- Resistor7/RConn1
  Controlled Voltage Source2/LConn1 -- Op-Amp3/LConn1
  Resistor10/RConn1 -- GND/RConn1 -- Voltage Sensor/RConn2 -- Op-Amp2/LConn1 -- Controlled Voltage Source2/RConn2
  Resistor9/LConn1 -- Resistor5/LConn1 -- Op-Amp4/LConn2
  Op-Amp4/RConn1 -- Voltage Sensor/LConn1 -- Resistor9/RConn1
  Resistor5/RConn1 -- Op-Amp2/LConn2 -- Resistor6/LConn1 -- Op-Amp2/RConn1
  Op-Amp3/RConn1 -- Op-Amp3/LConn2 -- Resistor6/RConn1 -- Resistor7/LConn1
  Controlled Voltage Source2/RConn1 -- IN/RConn1
  Vref/RConn1 -- PS-Simulink Converter/LConn1
  PS-Simulink Converter1/LConn1 -- Voltage Sensor/RConn1
  Simulink-PS Converter/RConn1 -- OUT/RConn1

== matlab function untitled/Sensor Humedad + Temperatura/i2c adapter ==
  data: data input; Temp_V output; T_min input; T_max input; RH_min input; RH_max input; Humi_V output
function [Temp_V, Humi_V] = ...
    i2c_to_digital(data, T_min,T_max,RH_min,RH_max)
%#codegen
% data: 1x6 uint8 = [T_MSB T_LSB CRC_T RH_MSB RH_LSB CRC_RH]
Temp_V=0.0; Humi_V=0.0; code8_T=uint8(0); code8_RH=uint8(0);

% Fuerza tamaño/tipo esperado (defensivo)
T_MSB=data(1); T_LSB=data(2); % CRC_T=data(3);
RH_MSB=data(4); RH_LSB=data(5); % CRC_RH=data(6);

rawT  = bitor(bitshift(uint16(T_MSB),8), uint16(T_LSB));
rawRH = bitor(bitshift(uint16(RH_MSB),8), uint16(RH_LSB));

T_C    = -45.0 + 175.0 * double(rawT)  / 65535.0;
RH_pct =  -6.0 + 125.0 * double(rawRH) / 65535.0;

dT  = T_max  - T_min; if dT  <= 0.0, dT  = 1.0; end
dRH = RH_max - RH_min; if dRH <= 0.0, dRH = 1.0; end

nT  = (T_C   - T_min)  / dT;   if nT  < 0.0, nT  = 0.0; elseif nT  > 1.0, nT  = 1.0; end
nRH = (RH_pct - RH_min)/ dRH;  if nRH < 0.0, nRH = 0.0; elseif nRH > 1.0, nRH = 1.0; end

code8_T  = uint8( round(255.0 * nT)  );
code8_RH = uint8( round(255.0 * nRH) );

Temp_V  = double(code8_T)  / 255.0;
Humi_V = double(code8_RH) / 255.0;

== matlab function untitled/Sensor Humedad + Temperatura/SHT45 ==
  data: T_C input; data output; RH_pct input
function data = SHT45(T_C, RH_pct)
%#codegen
% data: 1x6 uint8 SIEMPRE definido: [T_MSB T_LSB CRC_T RH_MSB RH_LSB CRC_RH]

% --- Preasigna vector fijo 1x6 uint8 (evita "undefined on some paths") ---
data = zeros(1,6,'uint8');

% --- Clamp entradas ---
T_C   = min(125.0, max(-40.0, double(T_C)));
RH_pct= min(100.0, max(0.0,   double(RH_pct)));

% --- Raw 16-bit ---
rawT  = uint16(round((T_C + 45.0)  / 175.0 * 65535.0));
rawRH = uint16(round((RH_pct + 6.0)/ 125.0 * 65535.0));

tmsb = uint8(bitshift(rawT,-8));  tlsb = uint8(bitand(rawT,255));
rhmsb= uint8(bitshift(rawRH,-8)); rhlsb= uint8(bitand(rawRH,255));

crcT  = local_crc8(tmsb, tlsb);
crcRH = local_crc8(rhmsb, rhlsb);

% --- Ensambla estrictamente 1x6 ---
data(1) = tmsb; data(2) = tlsb; data(3) = crcT;
data(4) = rhmsb; data(5) = rhlsb; data(6) = crcRH;

function c = local_crc8(b1,b2)
c    = uint8(255); poly = uint8(49);
c = bitxor(c,b1);
for k=1:8
    if bitand(c,uint8(128))~=0, c=bitxor(bitshift(c,1),poly); else, c=bitshift(c,1); end
    c = uint8(bitand(c,uint8(255)));
end
c = bitxor(c,b2);
for k=1:8
    if bitand(c,uint8(128))~=0, c=bitxor(bitshift(c,1),poly); else, c=bitshift(c,1); end
    c = uint8(bitand(c,uint8(255)));
end
end
end

== matlab function untitled/MATLAB Function ==
  settings: updateMethod=DISCRETE
  data: curr_in input; volt_in input; hum_in input; temp_in input; pinTemp output; pinHum output; pinVolt output; pinCurr output
function [   pinTemp, pinHum, pinVolt, pinCurr] = fcn(curr_in, volt_in, hum_in, temp_in)
%#codegen

persistent buffer count
if isempty(buffer)
    buffer = zeros(20,4); % 20 samples per second, 4 sensors
    count = 0;
end

% add newest sample
count = count + 1;
idx = mod(count-1,20) + 1;
buffer(idx,:) = [temp_in, hum_in, volt_in, curr_in];

% compute mean every 20 samples (~1 second)
if mod(count,20)==0
    cleanVals = mean(buffer,1);
else
    if count == 1
        cleanVals = buffer(idx,:); 
    else
        cleanVals = mean(buffer,1);
    end
end

% scale back to real units
temp_val = cleanVals(1)/3.3 * (125 - (-40)) + (-40);   % °C
hum_val  = cleanVals(2)/3.3 * 100;                     % %
volt_val = cleanVals(3)/3.3 * 1000;                    % V
curr_val = cleanVals(4)/3.3 * 100;                     % A

% digital danger flags (0 or 1)
pinTemp = double(temp_val > 10);
pinHum  = double(hum_val  > 60);
pinVolt = double(volt_val > 220);
pinCurr = double(curr_val > 50);
end

== matlab function untitled/Subsystem2/MATLAB Function ==
  settings: updateMethod=DISCRETE
  data: time input; regionAvgTemp input; T output; weatherCode input; H output
function [T, H] = WeatherModel(time, regionAvgTemp, weatherCode)
%#codegen
% Weather model with daily and weekly variation, no randomness

% ---- Time scaling ----
hour = mod(time,24);                % Hour of day [0,24)
weekPhase = mod(time,168)/168*2*pi; % Weekly cycle [0..2π]

% ---- Base amplitudes depending on weather ----
switch weatherCode
    case 0 % Sunny
        T_amp_day = 10;   % °C variation in a day
        H_base = 45;
    case 1 % Cloudy
        T_amp_day = 6;
        H_base = 60;
    case 2 % Rainy
        T_amp_day = 4;
        H_base = 80;
    otherwise
        T_amp_day = 7;
        H_base = 55;
end

% ---- Daily cycle (coldest ~6h, hottest ~15h) ----
dailyCycle = sin((hour-6)/24*2*pi);  

% ---- Weekly cycle (simulate warmer/cooler days) ----
weeklyCycle = 3 * sin(weekPhase);   % ±3°C across a week

% ---- Temperature ----
T = regionAvgTemp ...
    + T_amp_day * dailyCycle ...   % day/night swing
    + weeklyCycle;                 % weekly trend

% ---- Humidity ----
% Higher when temperature is low, lower when hot
H = H_base ...
    - 0.7*T_amp_day * dailyCycle ...  % anti-phase with temperature
    + 10*sin(weekPhase + pi/3);       % weekly humidity trend

% ---- Clamp to realistic ranges ----
T = max(min(T, 120), -40);      % -40..120°C

% Scale humidity to 0–1
H = max(min(H/100, 1), 0);      % 0..1 normalized
